simulink model "disturb"  (R2016a)
settings: Solver=VariableStepAuto  StartTime=0.0  StopTime=400  RelTol=1e-3
settings Model: Creator=xin  LastModifiedBy=xin

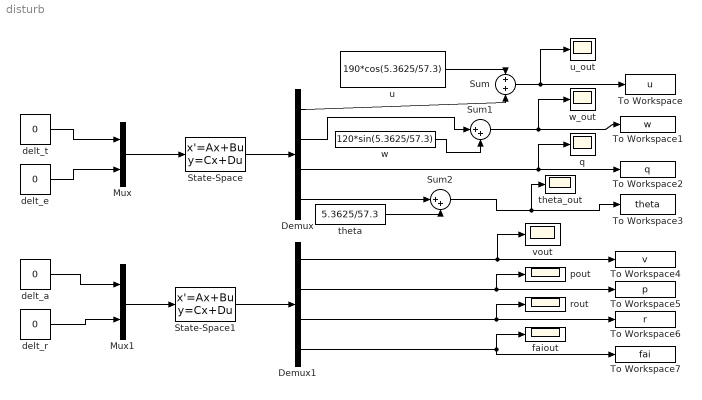
== system disturb ==
  Demux : Demux
  Demux1 : Demux
  Mux : Mux  Inputs=2
  Mux1 : Mux  Inputs=2
  State-Space : StateSpace  A=|  B=|  C=[1 0 0 0;0 1 0 0;0 0 1 0;0 0 0 1]  D=[0 0;0 0;0 0;0 0]  X0=[-0.0507 0.9973 -0.00009034 0.0007]
      A=|
      | [-0.00965935929732080	0.0369840269784605	0.283311074727651	-9.73308260370071;
      | -0.102903878346184	-0.422445640236601	182.819259963972	-0.913622921221361;
      | -3.22311254514824e-06	-0.000119526616308189	-0.452040286052541	0;
      | 0	0	1	0]
      B=|
      | [5.27116379592484	-0.000192464793591287;
      | 0	-0.168532156958147
      | ;0	-0.0933597179368480;
      | 0	0]
  State-Space1 : StateSpace  A=|  B=|  C=[1 0 0 0;0 1 0 0; 0 0 1 0; 0 0 0 1]  D=[0 0 ; 0 0 ;0 0 ;0 0 ]  X0=[0.9989; -0.025; 0.004 ;0.0158]
      A=|
      | [-0.133742123350947	0.0670499317885129	-189.484027251245	9.73308260370071;
      | -0.106749469992986	-1.48755186790463	0.399998266574683	0;
      | 0.0215189406635620	-0.0238598201074520	-0.200157981320062	0
      | ;0	1	0.0938677866428447	0]
      B=|
      | [0.0232840480007971	0.0635691469228112
      | ;-7.62685051510270	1.94638070253618;
      | -0.315501574261104	-0.960451844576626;
      | 0	0]
  Sum : Sum  Inputs=2
  Sum1 : Sum  Inputs=|++
  Sum2 : Sum  Inputs=|++
  To Workspace : ToWorkspace  VariableName=u  SaveFormat=Timeseries  SampleTime=-1
  To Workspace1 : ToWorkspace  VariableName=w  SaveFormat=Timeseries  SampleTime=-1
  To Workspace2 : ToWorkspace  VariableName=q  SaveFormat=Timeseries  SampleTime=-1
  To Workspace3 : ToWorkspace  VariableName=theta  SaveFormat=Timeseries  SampleTime=-1
  To Workspace4 : ToWorkspace  VariableName=v  SaveFormat=Timeseries  SampleTime=-1
  To Workspace5 : ToWorkspace  VariableName=p  SaveFormat=Timeseries  SampleTime=-1
  To Workspace6 : ToWorkspace  VariableName=r  SaveFormat=Timeseries  SampleTime=-1
  To Workspace7 : ToWorkspace  VariableName=fai  SaveFormat=Timeseries  SampleTime=-1
  delt_a : Constant  Value=0
  delt_e : Constant  Value=0
  delt_r : Constant  Value=0
  delt_t : Constant  Value=0
  faiout : Scope
  pout : Scope
  q : Scope
  rout : Scope
  theta : Constant  Value=5.3625/57.3
  theta_out : Scope
  u : Constant  Value=190*cos(5.3625/57.3)
  "u_out " : Scope
  vout : Scope
  w : Constant  Value=120*sin(5.3625/57.3)
  w_out : Scope
  wires:
  delt_t/1 -> Mux/1
  delt_e/1 -> Mux/2
  Mux/1 -> State-Space/1
  delt_a/1 -> Mux1/1
  delt_r/1 -> Mux1/2
  Mux1/1 -> State-Space1/1
  State-Space/1 -> Demux/1
  State-Space1/1 -> Demux1/1
  Demux/1 -> Sum/2
  u/1 -> Sum/1
  Sum/1 -> To Workspace/1, "u_out "/1
  Demux/2 -> Sum1/1
  w/1 -> Sum1/2
  Sum1/1 -> To Workspace1/1, w_out/1
  Demux/3 -> q/1, To Workspace2/1
  Demux/4 -> Sum2/1
  theta/1 -> Sum2/2
  Sum2/1 -> theta_out/1, To Workspace3/1
  Demux1/1 -> vout/1, To Workspace4/1
  Demux1/2 -> pout/1, To Workspace5/1
  Demux1/3 -> rout/1, To Workspace6/1
  Demux1/4 -> faiout/1, To Workspace7/1
